simulink model "KR6_InverseKinematics"  (R2018a)
settings: Solver=VariableStepAuto  StartTime=0.0  StopTime=inf  RelTol=1e-3
libraries: vrlib x8, KR6_Lib x2, dspindex x1
settings Model: Creator=Pedro Ramalho  LastModifiedBy=Pedro Ramalho

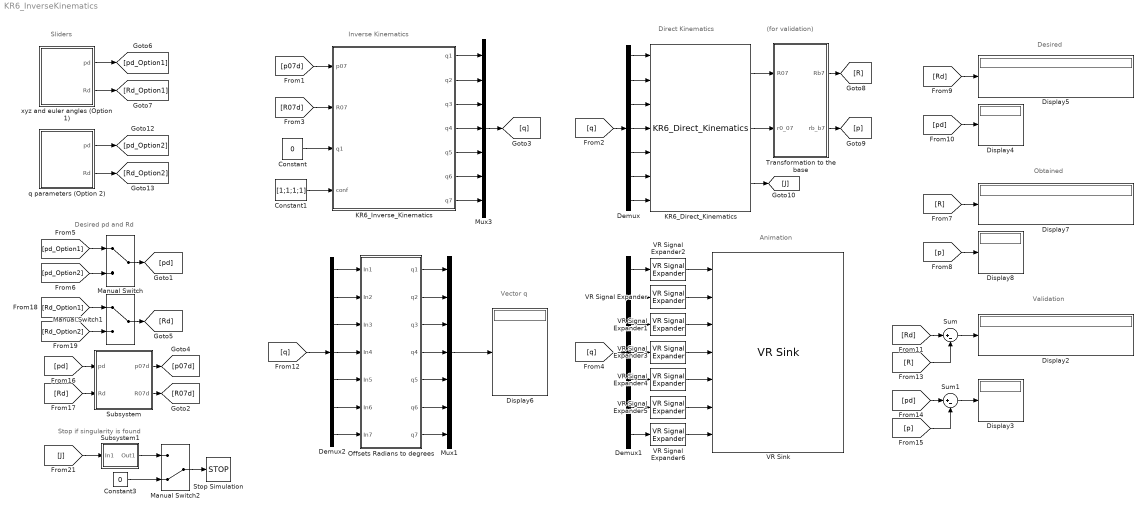
== system KR6_InverseKinematics ==
  note: Sliders
  note: Animation
  note: Direct Kinematics
  note: Inverse Kinematics
  note: Validation
  note: Vector q
  note: Desired
  note: Obtained
  note: Desired pd and Rd
  note: (for validation)
  note: Stop if singularity is found
  Constant : Constant  Value=0
  Constant1 : Constant  Value=[1;1;1;1]
  Constant3 : Constant  Value=0
  Demux : Demux  Outputs=7
  Demux1 : Demux  Outputs=7
  Demux2 : Demux  Outputs=7
  Display{2..8} (7 alike) : Display
  KR6_Direct_Kinematics : KR6_Lib/KR6_Direct_Kinematics
  KR6_Inverse_Kinematics : MATLAB Function  TreatAsAtomicUnit=on
  Manual Switch : ManualSwitch
  Manual Switch1 : ManualSwitch
  Manual Switch2 : ManualSwitch  CurrentSetting=0
  Mux1 : Mux  Inputs=7
  Mux3 : Mux  Inputs=7
  Offsets Radians to degrees : Subsystem
  Stop Simulation : Stop
  Subsystem : Subsystem
  Subsystem1 : Subsystem
  Sum : Sum  Inputs=|+-
  Sum1 : Sum  Inputs=|+-
  Transformation to the base : Subsystem
  VR Signal Expander{,1,3..6} (6 alike) : vrlib/VR Signal Expander  outwidth=4  outidx=4
      settings: SourceProductName=Simulink 3D Animation  SourceProductBaseCode=VR
  VR Signal Expander2 : vrlib/VR Signal Expander  outwidth=3  outidx=3
      settings: SourceProductName=Simulink 3D Animation  SourceProductBaseCode=VR
  VR Sink : vrlib/VR Sink  InstantiateOnLoad=on  SampleTime=0.1  ViewEnable=on  RemoteChange=off  RemoteView=off  FieldsWritten=Jt1_DH_dv.translation.3.1.1.double#Jt2_DH_dv.rotation.4.1.1.double#Jt3_DH_dv.rotation.4.1.1.double#Jt4_DH_dv.rotation.4.1.1.double#Jt5_DH_dv.rotation.4.1.1.double#Jt6_DH_dv.rotation.4.1.1.double#Jt7_DH_dv.rotation.4.1.1.double  WorldFileName=vrrobotKR6.wrl  WorldDescription=D-H Reference Frames for Virtual Reality Robot  AutoView=off  VideoDimensions=[]  AllowVariableSize=off
      settings: SourceProductBaseCode=VR
  q parameters (Option 2) : Subsystem  mask{q1=0.3, q2=45.01, q3=-45, q4=45, q5=45.07, q6=45.05, q7=45}
  xyz and euler angles (Option 1) : Subsystem  mask{px=0, py=0.470, pz=1.106, phi=0, theta=90, psi=-90}
      mask prompts: px "x"; py "y"; pz "z"
      mask DialogControl ParameterGroupVar_copy Prompt: Euler angles
  wires:
  VR Signal Expander2/1 -> VR Sink/1
  VR Signal Expander/1 -> VR Sink/2
  VR Signal Expander1/1 -> VR Sink/3
  VR Signal Expander3/1 -> VR Sink/4
  VR Signal Expander4/1 -> VR Sink/5
  VR Signal Expander5/1 -> VR Sink/6
  VR Signal Expander6/1 -> VR Sink/7
  KR6_Direct_Kinematics/3 -> [J]
  Demux/1 -> KR6_Direct_Kinematics/1
  Demux/2 -> KR6_Direct_Kinematics/2
  Demux/3 -> KR6_Direct_Kinematics/3
  Demux/4 -> KR6_Direct_Kinematics/4
  Demux/5 -> KR6_Direct_Kinematics/5
  Demux/6 -> KR6_Direct_Kinematics/6
  Demux/7 -> KR6_Direct_Kinematics/7
  [q] -> Demux/1
  [q] -> Demux1/1
  Demux1/1 -> VR Signal Expander2/1
  Demux1/3 -> VR Signal Expander1/1
  Demux1/6 -> VR Signal Expander5/1
  Demux1/2 -> VR Signal Expander/1
  Demux1/5 -> VR Signal Expander4/1
  Demux1/4 -> VR Signal Expander3/1
  Demux1/7 -> VR Signal Expander6/1
  KR6_Inverse_Kinematics/1(q1) -> Mux3/1
  KR6_Inverse_Kinematics/2(q2) -> Mux3/2
  KR6_Inverse_Kinematics/3(q3) -> Mux3/3
  KR6_Inverse_Kinematics/4(q4) -> Mux3/4
  KR6_Inverse_Kinematics/5(q5) -> Mux3/5
  KR6_Inverse_Kinematics/6(q6) -> Mux3/6
  KR6_Inverse_Kinematics/7(q7) -> Mux3/7
  Mux3/1 -> [q]
  [R07d] -> KR6_Inverse_Kinematics/2(R07)
  [p07d] -> KR6_Inverse_Kinematics/1(p07)
  Constant/1 -> KR6_Inverse_Kinematics/3("q1 ")
  [q] -> Demux2/1
  Demux2/4 -> Offsets Radians to degrees/4(In4)
  Mux1/1 -> Display6/1
  Demux2/6 -> Offsets Radians to degrees/6(In6)
  Offsets Radians to degrees/1(q1) -> Mux1/1
  Offsets Radians to degrees/4(q4) -> Mux1/4
  Demux2/7 -> Offsets Radians to degrees/7(In7)
  Demux2/1 -> Offsets Radians to degrees/1(In1)
  Offsets Radians to degrees/2(q2) -> Mux1/2
  Demux2/5 -> Offsets Radians to degrees/5(In5)
  Demux2/3 -> Offsets Radians to degrees/3(In3)
  Offsets Radians to degrees/5(q5) -> Mux1/5
  Offsets Radians to degrees/7(q7) -> Mux1/7
  Offsets Radians to degrees/3(q3) -> Mux1/3
  Demux2/2 -> Offsets Radians to degrees/2(In2)
  Offsets Radians to degrees/6(q6) -> Mux1/6
  KR6_Direct_Kinematics/1 -> Transformation to the base/1(R07)
  KR6_Direct_Kinematics/2 -> Transformation to the base/2(r0_07)
  Transformation to the base/1(Rb7) -> [R]
  Constant1/1 -> KR6_Inverse_Kinematics/4(conf)
  [R] -> Display7/1
  [p] -> Display8/1
  xyz and euler angles (Option 1)/1(pd) -> [pd_Option1]
  xyz and euler angles (Option 1)/2(Rd) -> [Rd_Option1]
  [Rd] -> Display5/1
  [pd] -> Display4/1
  Transformation to the base/2(rb_b7) -> [p]
  [Rd] -> Sum/1
  [R] -> Sum/2
  Sum/1 -> Display2/1
  Sum1/1 -> Display3/1
  [pd] -> Sum1/1
  [p] -> Sum1/2
  [pd_Option2] -> Manual Switch/2
  [pd_Option1] -> Manual Switch/1
  Manual Switch/1 -> [pd]
  [pd] -> Subsystem/1(pd)
  Subsystem/2(R07d) -> [R07d]
  Subsystem/1(p07d) -> [p07d]
  [Rd] -> Subsystem/2(Rd)
  [Rd_Option1] -> Manual Switch1/1
  Manual Switch1/1 -> [Rd]
  [Rd_Option2] -> Manual Switch1/2
  q parameters (Option 2)/1(pd) -> [pd_Option2]
  q parameters (Option 2)/2(Rd) -> [Rd_Option2]
  Constant3/1 -> Manual Switch2/2
  Manual Switch2/1 -> Stop Simulation/1
  [J] -> Subsystem1/1(In1)
  Subsystem1/1(Out1) -> Manual Switch2/1

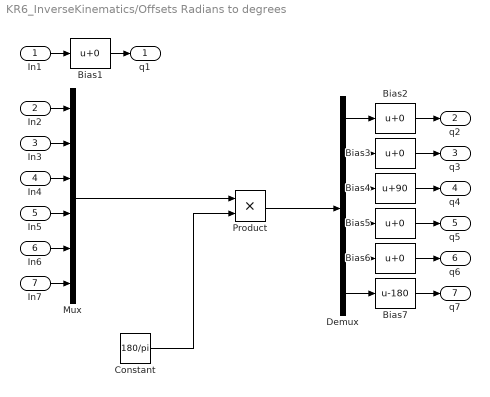
== system KR6_InverseKinematics/Offsets Radians to degrees ==
  In1 : Inport
  In2 : Inport  Port=2
  In3 : Inport  Port=3
  In4 : Inport  Port=4
  In5 : Inport  Port=5
  In6 : Inport  Port=6
  In7 : Inport  Port=7
  Bias{1..3,5..6} (5 alike) : Bias
  Bias4 : Bias  Bias=90
  Bias7 : Bias  Bias=-180
  Constant : Constant  Value=180/pi
  Demux : Demux  Outputs=6
  Mux : Mux  Inputs=6
  Product : Product
  q1 : Outport
  q2 : Outport  Port=2
  q3 : Outport  Port=3
  q4 : Outport  Port=4
  q5 : Outport  Port=5
  q6 : Outport  Port=6
  q7 : Outport  Port=7
  wires:
  In1/1 -> Bias1/1
  Bias1/1 -> q1/1
  Mux/1 -> Product/1
  Constant/1 -> Product/2
  Product/1 -> Demux/1
  In2/1 -> Mux/1
  In3/1 -> Mux/2
  In4/1 -> Mux/3
  In5/1 -> Mux/4
  In6/1 -> Mux/5
  In7/1 -> Mux/6
  Demux/1 -> Bias2/1
  Demux/2 -> Bias3/1
  Demux/3 -> Bias4/1
  Demux/4 -> Bias5/1
  Demux/5 -> Bias6/1
  Demux/6 -> Bias7/1
  Bias2/1 -> q2/1
  Bias3/1 -> q3/1
  Bias4/1 -> q4/1
  Bias5/1 -> q5/1
  Bias6/1 -> q6/1
  Bias7/1 -> q7/1

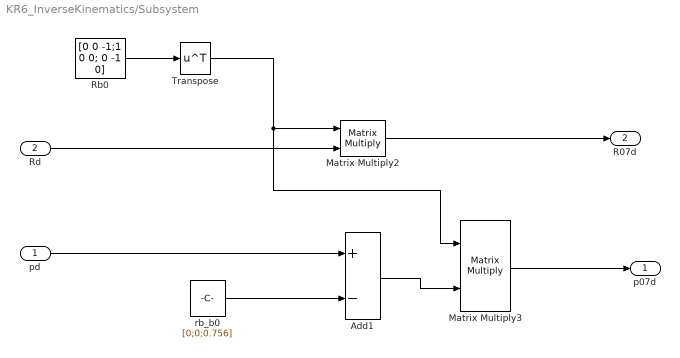
== system KR6_InverseKinematics/Subsystem ==
  pd : Inport
  Rd : Inport  Port=2
  Add1 : Sum  Inputs=+-
  Matrix Multiply2 : Product  Multiplication=Matrix(*)
  Matrix Multiply3 : Product  Multiplication=Matrix(*)
  Rb0 : Constant  Value=[0 0 -1;1 0 0; 0 -1 0]
  Transpose : Math  Operator=transpose  SaturateOnIntegerOverflow=on
  rb_b0 : Constant  Value=[0;0;0.756]
  p07d : Outport
  R07d : Outport  Port=2
  wires:
  Add1/1 -> Matrix Multiply3/2
  Matrix Multiply3/1 -> p07d/1
  Rb0/1 -> Transpose/1
  Transpose/1 -> Matrix Multiply3/1, Matrix Multiply2/1
  Rd/1 -> Matrix Multiply2/2
  rb_b0/1 -> Add1/2
  pd/1 -> Add1/1
  Matrix Multiply2/1 -> R07d/1

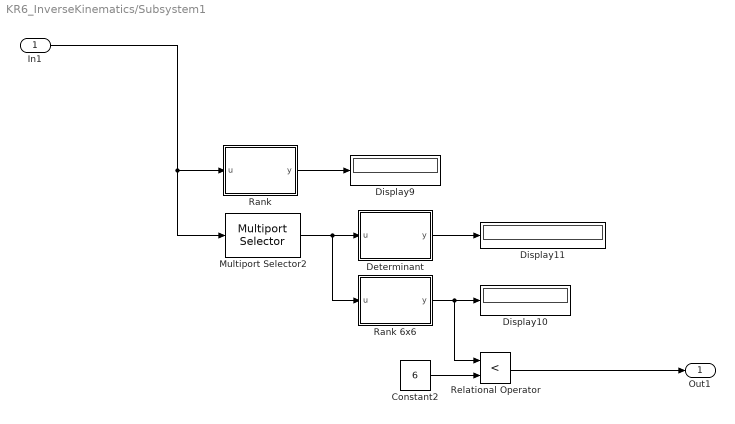
== system KR6_InverseKinematics/Subsystem1 ==
  In1 : Inport
  " Determinant" : MATLAB Function  TreatAsAtomicUnit=on
  Constant2 : Constant  Value=6
  Display10 : Display
  Display11 : Display
  Display9 : Display
  Multiport Selector2 : dspindex/Multiport Selector  rowsOrCols=Columns  idxCellArray={[2:7]}  idxErrMode=Clip Index
  Rank : MATLAB Function  TreatAsAtomicUnit=on
  Rank 6x6 : MATLAB Function  TreatAsAtomicUnit=on
  Relational Operator : RelationalOperator  Operator=<  OutDataTypeStr=boolean  RndMeth=Simplest
  Out1 : Outport
  wires:
  Rank 6x6/1(y) -> Relational Operator/1, Display10/1
  In1/1 -> Multiport Selector2/1, Rank/1(u)
  Multiport Selector2/1 -> Rank 6x6/1(u), " Determinant"/1(u)
  Relational Operator/1 -> Out1/1
  Constant2/1 -> Relational Operator/2
  " Determinant"/1(y) -> Display11/1
  Rank/1(y) -> Display9/1

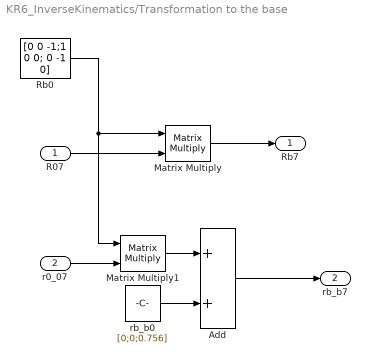
== system KR6_InverseKinematics/Transformation to the base ==
  R07 : Inport
  r0_07 : Inport  Port=2
  Add : Sum
  Matrix Multiply : Product  Multiplication=Matrix(*)
  Matrix Multiply1 : Product  Multiplication=Matrix(*)
  Rb0 : Constant  Value=[0 0 -1;1 0 0; 0 -1 0]
  rb_b0 : Constant  Value=[0;0;0.756]
  Rb7 : Outport
  rb_b7 : Outport  Port=2
  wires:
  Matrix Multiply1/1 -> Add/1
  R07/1 -> Matrix Multiply/2
  rb_b0/1 -> Add/2
  Rb0/1 -> Matrix Multiply1/1, Matrix Multiply/1
  Matrix Multiply/1 -> Rb7/1
  r0_07/1 -> Matrix Multiply1/2
  Add/1 -> rb_b7/1

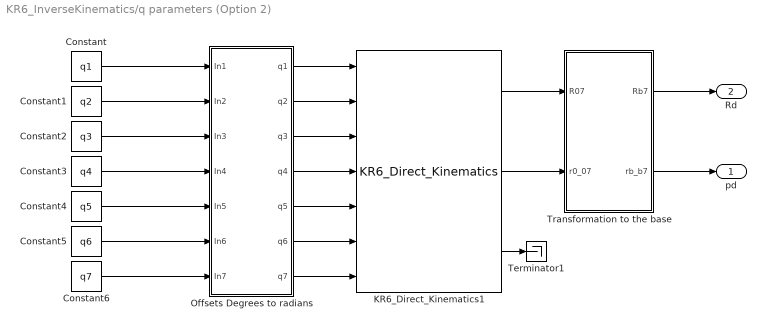
== system KR6_InverseKinematics/q parameters (Option 2) ==
  Constant : Constant  Value=q1
  Constant1 : Constant  Value=q2
  Constant2 : Constant  Value=q3
  Constant3 : Constant  Value=q4
  Constant4 : Constant  Value=q5
  Constant5 : Constant  Value=q6
  Constant6 : Constant  Value=q7
  KR6_Direct_Kinematics1 : KR6_Lib/KR6_Direct_Kinematics
  Offsets Degrees to radians : Subsystem
  Terminator1 : Terminator
  Transformation to the base : Subsystem
  pd : Outport
  Rd : Outport  Port=2
  wires:
  Transformation to the base/2(rb_b7) -> pd/1
  KR6_Direct_Kinematics1/2 -> Transformation to the base/2(r0_07)
  Constant3/1 -> Offsets Degrees to radians/4(In4)
  Transformation to the base/1(Rb7) -> Rd/1
  Constant4/1 -> Offsets Degrees to radians/5(In5)
  KR6_Direct_Kinematics1/1 -> Transformation to the base/1(R07)
  Constant2/1 -> Offsets Degrees to radians/3(In3)
  Constant5/1 -> Offsets Degrees to radians/6(In6)
  KR6_Direct_Kinematics1/3 -> Terminator1/1
  Constant6/1 -> Offsets Degrees to radians/7(In7)
  Constant1/1 -> Offsets Degrees to radians/2(In2)
  Constant/1 -> Offsets Degrees to radians/1(In1)
  Offsets Degrees to radians/1(q1) -> KR6_Direct_Kinematics1/1
  Offsets Degrees to radians/2(q2) -> KR6_Direct_Kinematics1/2
  Offsets Degrees to radians/3(q3) -> KR6_Direct_Kinematics1/3
  Offsets Degrees to radians/4(q4) -> KR6_Direct_Kinematics1/4
  Offsets Degrees to radians/5(q5) -> KR6_Direct_Kinematics1/5
  Offsets Degrees to radians/6(q6) -> KR6_Direct_Kinematics1/6
  Offsets Degrees to radians/7(q7) -> KR6_Direct_Kinematics1/7

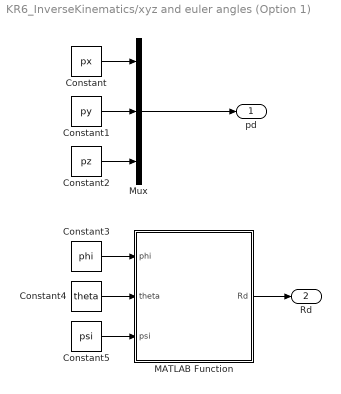
== system KR6_InverseKinematics/xyz and euler angles (Option 1) ==
  Constant : Constant  Value=px
  Constant1 : Constant  Value=py
  Constant2 : Constant  Value=pz
  Constant3 : Constant  Value=phi
  Constant4 : Constant  Value=theta
  Constant5 : Constant  Value=psi
  MATLAB Function : MATLAB Function  TreatAsAtomicUnit=on
  Mux : Mux  Inputs=3
  pd : Outport
  Rd : Outport  Port=2
  wires:
  Constant/1 -> Mux/1
  Constant1/1 -> Mux/2
  Constant2/1 -> Mux/3
  Mux/1 -> pd/1
  Constant3/1 -> MATLAB Function/1(phi)
  Constant4/1 -> MATLAB Function/2(theta)
  Constant5/1 -> MATLAB Function/3(psi)
  MATLAB Function/1(Rd) -> Rd/1

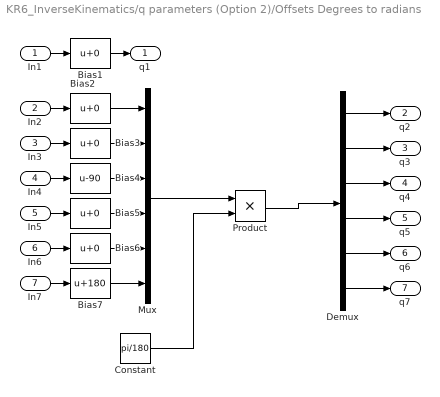
== system KR6_InverseKinematics/q parameters (Option 2)/Offsets Degrees to radians ==
  In1 : Inport
  In2 : Inport  Port=2
  In3 : Inport  Port=3
  In4 : Inport  Port=4
  In5 : Inport  Port=5
  In6 : Inport  Port=6
  In7 : Inport  Port=7
  Bias{1..3,5..6} (5 alike) : Bias
  Bias4 : Bias  Bias=-90
  Bias7 : Bias  Bias=180
  Constant : Constant  Value=pi/180
  Demux : Demux  Outputs=6
  Mux : Mux  Inputs=6
  Product : Product
  q1 : Outport
  q2 : Outport  Port=2
  q3 : Outport  Port=3
  q4 : Outport  Port=4
  q5 : Outport  Port=5
  q6 : Outport  Port=6
  q7 : Outport  Port=7
  wires:
  In6/1 -> Bias6/1
  In5/1 -> Bias5/1
  In3/1 -> Bias3/1
  In1/1 -> Bias1/1
  Bias1/1 -> q1/1
  In7/1 -> Bias7/1
  In4/1 -> Bias4/1
  In2/1 -> Bias2/1
  Bias7/1 -> Mux/6
  Bias2/1 -> Mux/1
  Bias3/1 -> Mux/2
  Bias4/1 -> Mux/3
  Bias5/1 -> Mux/4
  Bias6/1 -> Mux/5
  Mux/1 -> Product/1
  Constant/1 -> Product/2
  Demux/1 -> q2/1
  Demux/2 -> q3/1
  Demux/3 -> q4/1
  Demux/4 -> q5/1
  Demux/5 -> q6/1
  Demux/6 -> q7/1
  Product/1 -> Demux/1

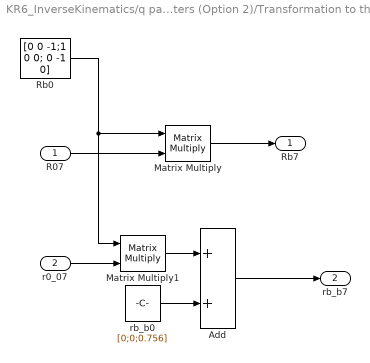
== system KR6_InverseKinematics/q parameters (Option 2)/Transformation to the base ==
  R07 : Inport
  r0_07 : Inport  Port=2
  Add : Sum
  Matrix Multiply : Product  Multiplication=Matrix(*)
  Matrix Multiply1 : Product  Multiplication=Matrix(*)
  Rb0 : Constant  Value=[0 0 -1;1 0 0; 0 -1 0]
  rb_b0 : Constant  Value=[0;0;0.756]
  Rb7 : Outport
  rb_b7 : Outport  Port=2
  wires:
  Matrix Multiply1/1 -> Add/1
  R07/1 -> Matrix Multiply/2
  rb_b0/1 -> Add/2
  Rb0/1 -> Matrix Multiply1/1, Matrix Multiply/1
  Matrix Multiply/1 -> Rb7/1
  r0_07/1 -> Matrix Multiply1/2
  Add/1 -> rb_b7/1

== matlab function KR6_InverseKinematics/KR6_Inverse_Kinematics ==
  data: p07 input; R07 input; q1 output; q2 output; q3 output; q4 output; q5 output; q6 output; q7 output; q1 input; conf input
function [q1,q2,q3,q4,q5,q6,q7]  = KR6_Inverse_Kinematics(p07,R07,q1,conf)
%conf: robot configuration
%conf(1): elbow up: 1
%         elbow down: 0
%conf(2): wrist I: 1
%         wrist II: 0
%conf(3): facing forward: 1
%         facing backward: 0
%conf(4): q1 fixed: 1
%         q1 not fixed: 0 (equal to position x from base reference frame)

q1 = q1*conf(4) + p07(3) *(1-conf(4));


a2 =25*10^-3;
a3 = 315*10^-3;
a4 =35*10^-3;
d5 =-365*10^-3;
d7 = -80*10^-3;


%% q2
pw = p07 + d7 * R07(:,3) -[0;0;q1];

q2FW = - atan2(pw(3),pw(1));
q2BW = - atan2(pw(3),pw(1)) + pi;
q2 = q2FW*conf(3) + q2BW*(1-conf(3));

%% q4
aw = (a4^2 + d5^2)^0.5;

%l^2 = wy^2 + ((wx^2+wz^2)^0.5-a2)^2
lFW = ( pw(2)^2 + ((pw(1)^2+pw(3)^2)^0.5 -a2)^2)^0.5;
lBW = ( pw(2)^2 + ((pw(1)^2+pw(3)^2)^0.5 +a2)^2)^0.5;
l = lFW*conf(3) + lBW*(1-conf(3));

cw = (l^2 - a3^2 - aw^2)/(2*a3*aw);
sw = (1-cw^2)^0.5;
thetaw = atan2(sw,cw);
gama = atan(-d5/a4);

q4FW = (thetaw-gama)*conf(1) - (thetaw + gama)*(1-conf(1));
q4BW = - (thetaw + gama)*conf(1) + (thetaw-gama)*(1-conf(1));
q4 = q4FW*conf(3) + q4BW*(1-conf(3));

%% q3
%alfa = arctg(-wy,(wx^2+wz^2)^0.5-a2)
alfaFW = atan2(-pw(2),(pw(1)^2+pw(3)^2)^0.5 -a2);
alfaBW = atan2(-pw(2),(pw(1)^2+pw(3)^2)^0.5 +a2);
alfa = alfaFW*conf(3) + alfaBW*(1-conf(3));

%beta = arctg(aw(1-cw^2)^0.5,a3+aw*cw)
beta = atan2(aw*(1-cw^2)^0.5,a3+aw*cw);

q3FW = (-alfa-beta)*conf(1) + (-alfa+beta)*(1-conf(1));
q3BW = (beta+alfa-pi)*conf(1) + (pi+alfa-beta)*(1-conf(1));
q3 = q3FW*conf(3) + q3BW*(1-conf(3));

%% Computing q5,q6 and q7
R04 = [cos(q3 + q4)*cos(q2), sin(q2),  sin(q3 + q4)*cos(q2);
       sin(q3 + q4),       0,         -cos(q3 + q4);
      -cos(q3 + q4)*sin(q2), cos(q2), -sin(q3 + q4)*sin(q2)];
 
R47 = R04'*R07;

%R47: %Symbolic expression
%[ cos(q5)*cos(q6)*cos(q7) - sin(q5)*sin(q7), cos(q7)*sin(q5) + cos(q5)*cos(q6)*sin(q7), -cos(q5)*sin(q6)]
%[ cos(q5)*sin(q7) + cos(q6)*cos(q7)*sin(q5), cos(q6)*sin(q5)*sin(q7) - cos(q5)*cos(q7), -sin(q5)*sin(q6)]
%[                          -cos(q7)*sin(q6),                          -sin(q6)*sin(q7),         -cos(q6)]

%Wrist configuration I: (conf(2) = 1)
q5I = atan2(-R47(2,3),-R47(1,3));
q6I = atan2((R47(3,1)^2+R47(3,2)^2)^0.5,-R47(3,3));
q7I = atan2(-R47(3,2),-R47(3,1))+2*pi;

%Wrist configuration II: (conf(2) = 0)
q5II = atan2(R47(2,3),R47(1,3));
q6II = atan2(-(R47(3,1)^2+R47(3,2)^2)^0.5,-R47(3,3));
q7II = atan2(R47(3,2),R47(3,1));

q5 = q5I*conf(2) + q5II*(1-conf(2));
q6 = q6I*conf(2) + q6II*(1-conf(2));
q7 = q7I*conf(2) + q7II*(1-conf(2));

== matlab function KR6_InverseKinematics/Subsystem1/ Determinant ==
  data: u input; y output
function y = fcn(u)

y = det(u);
%determinante do jacobiano

== matlab function KR6_InverseKinematics/xyz and euler angles (Option 1)/MATLAB Function ==
  data: phi input; Rd output; theta input; psi input
function Rd = fcn(phi,theta,psi)

eul = pi/180*[phi theta psi];
Rd = eul2rotm(eul);

end

== matlab function KR6_InverseKinematics/Subsystem1/Rank ==
  data: u input; y output
function y = fcn(u)

y = rank(u);
%rank do jacobiano

== matlab function KR6_InverseKinematics/Subsystem1/Rank 6x6 ==
  data: u input; y output
function y = fcn(u)

y = rank(u);
%rank do jacobiano
